simulink model "Dimmer"  (R2014a)
settings: Solver=ode15s  StartTime=0.0  StopTime=0.08  MaxStep=0.001  RelTol=1e-3
libraries: fl_lib x31, elec_lib x7, nesl_utility x4
Description:
  | Full-Wave Bridge Rectifier
  | 
  | This example shows an ideal AC transformer plus full-wave bridge rectifier.
  | It converts 120 volts AC to 12 volts DC. The transformer has a turns ratio
  | of 14, stepping the supply down to 8.6 volts rms, i.e. 8.6*sqrt(2) = 12 volts
  | pk-pk. The full-wave bridge rectifier plus capacitor combination
  | then converts this to DC. The resistor represents a typical load.
  | 
  | The model can be used to size the capacitor required for a specified load.
  | For a given size of capacitor, as the load resistance is increased, the ripple
  | in the DC voltage increases. The model can also be used to drive an
  | application circuit in order to assess the effect of the ripple.
  | 
  | 
  | 
  | 
  | Copyright 2008-2014 The MathWorks, Inc.
settings Model: ExtModeAutoUpdateStatusClock=off  Creator=MathWorks  LastModifiedBy=keelan
settings DataIOCC: SignalLoggingSaveFormat=ModelDataLogs
settings OptimizationCC: ExpressionDepthLimit=2147483647  InitFltsAndDblsToZero=on  EfficientMapNaN2IntZero=off
settings DebuggingCC: SaveWithParameterizedLinksMsg=none  UnderspecifiedInitializationDetection=Classic  SignalResolutionControl=TryResolveAllWithWarning  FcnCallInpInsideContextMsg=UseLocalSettings  StateNameClashWarn=warning
settings GRTTargetCC: TargetFcnLib=ansi_tfl_tmw.mat  CombineOutputUpdateFcns=off  GRTInterface=on
settings SimscapeCC: ExplicitSolverDiagnosticOptions=none

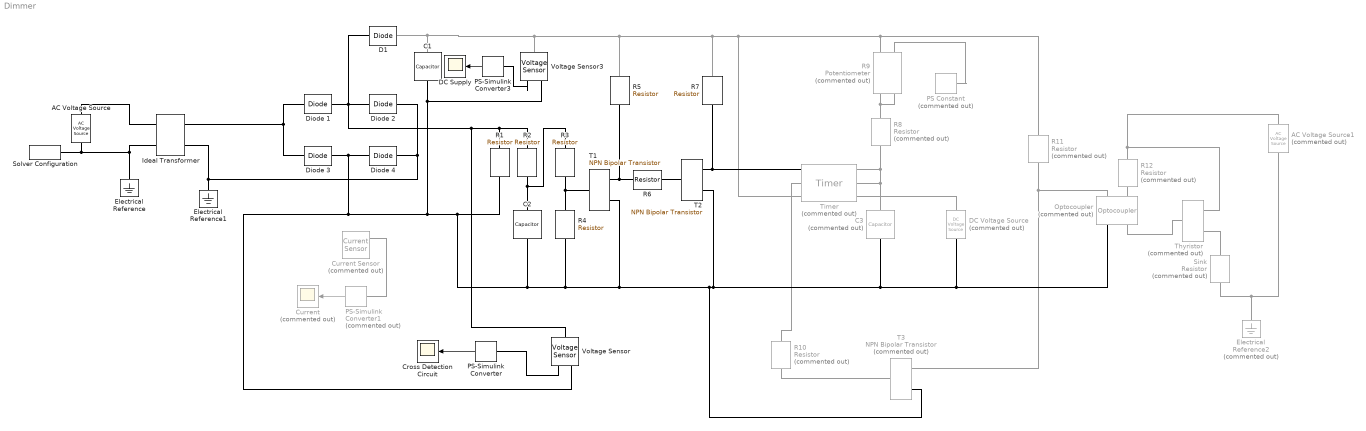
== system Dimmer ==
  AC Voltage Source : fl_lib/Electrical/Electrical Sources/AC Voltage Source  amp=240 V  shift=0 deg  frequency=50 Hz  omega=0 rad/s
  AC Voltage Source1 : fl_lib/Electrical/Electrical Sources/AC Voltage Source  Commented=on  amp=240 V  shift=0 deg  frequency=50 Hz  omega=0 rad/s
  C1 : fl_lib/Electrical/Electrical Elements/Capacitor  c=1000 uF  r=1e-06 Ohm  g=0 1/Ohm  i_specify=off  i_priority=High  i=0 A  v_specify=off  v_priority=High  v=0 V  vc_specify=on  vc_priority=High  vc=0 V
  C2 : fl_lib/Electrical/Electrical Elements/Capacitor  c=0.1 nF  r=1e-06 Ohm  g=0 1/Ohm  i_specify=off  i_priority=High  i=0 A  v_specify=off  v_priority=High  v=0 V  vc_specify=on  vc_priority=High  vc=0 V
  C3 : fl_lib/Electrical/Electrical Elements/Capacitor  Commented=on  c=1 uF  r=1e-06 Ohm  g=0 1/Ohm  i_specify=off  i_priority=High  i=0 A  v_specify=off  v_priority=High  v=0 V  vc_specify=on  vc_priority=High  vc=0 V
  Cross Detection Circuit : Scope
      settings: YMin=-0.25  YMax=3.5
  Current : Scope  Commented=on
      settings: YMin=-0.25  YMax=3.5
  Current Sensor : fl_lib/Electrical/Electrical Sensors/Current Sensor  Commented=on
  D1 : fl_lib/Electrical/Electrical Elements/Diode  Vf=0.1 V  Ron=0.1 Ohm  Goff=1e-8 1/Ohm  i_specify=off  i_priority=High  i=0 A  v_specify=off  v_priority=High  v=0 V
  DC Supply : Scope
      settings: TimeRange=10  YMin=-0.5  YMax=7.5  SaveName=ScopeData3
  DC Voltage Source : fl_lib/Electrical/Electrical Sources/DC Voltage Source  Commented=on  v0=0 V
  Diode {1..4} (4 alike) : fl_lib/Electrical/Electrical Elements/Diode  Vf=0.6 V  Ron=0.3 Ohm  Goff=1e-08 1/Ohm  i_specify=off  i_priority=High  i=0 A  v_specify=off  v_priority=High  v=0 V
  Electrical Reference : fl_lib/Electrical/Electrical Elements/Electrical Reference
  Electrical Reference1 : fl_lib/Electrical/Electrical Elements/Electrical Reference
  Electrical Reference2 : fl_lib/Electrical/Electrical Elements/Electrical Reference  Commented=on
  Ideal Transformer : fl_lib/Electrical/Electrical Elements/Ideal Transformer  n=26.666*2  i1_specify=off  i1_priority=High  i1=0 A  v1_specify=off  v1_priority=High  v1=0 V  i2_specify=off  i2_priority=High  i2=0 A  v2_specify=off  v2_priority=High  v2=0 V
  Optocoupler : elec_lib/Semiconductor Devices/Optocoupler  Commented=on  CTR=0.2  prmExp=1  I12=[ 0.001 0.015 ] A  V12=[ 0.9 1.05 ] V  RS=0.1 Ohm  IS=1e-10 A  Tmeas=25 C  ec=2  C_param=1  CJ0=5 pF  VJ=1 V  Mgrad=0.5  Vvec=[ 0.1 10 100 ] V  Cvec=[ 3.5 1 0.4 ] pF  FC=0.5  T_param=1  IS_T2=1.8e-8 A  I1_T2=0.029 A  V1_T2=1.05 V  Tmeas2=125 C  EG_param=1  EG=1.11 eV  XTI_param=1  XTI=3  Tdevice=25 C  Rth=[ 0 10 ] K/W  thermal_mass_parameterization=1  thermal_mass=[ 0 1 ] J/K  thermal_time_constant=[ 0 10 ] s  thermal_mass_initial_temperatures=[ 25 25 ] C
  PS Constant : fl_lib/Physical Signals/Sources/PS Constant  Commented=on  constant=1
  PS-Simulink Converter : nesl_utility/PS-Simulink Converter  PhysicalDomain=network_engine_domain  SubClassName=ps_output  LeftPortType=input  RightPortType=output  PseudoPeriodic=off  Frequencies=[]  Unit=1  AffineConversion=off
  PS-Simulink Converter1 : nesl_utility/PS-Simulink Converter  Commented=on  PhysicalDomain=network_engine_domain  SubClassName=ps_output  LeftPortType=input  RightPortType=output  PseudoPeriodic=off  Frequencies=[]  Unit=1  AffineConversion=off
  PS-Simulink Converter3 : nesl_utility/PS-Simulink Converter  PhysicalDomain=network_engine_domain  SubClassName=ps_output  LeftPortType=input  RightPortType=output  PseudoPeriodic=off  Frequencies=[]  Unit=1  AffineConversion=off
  R1 : fl_lib/Electrical/Electrical Elements/Resistor  R=10 kOhm  i_specify=off  i_priority=High  i=0 A  v_specify=off  v_priority=High  v=0 V
  R{8,10..12} (4 alike) : fl_lib/Electrical/Electrical Elements/Resistor  Commented=on  R=1 kOhm  i_specify=off  i_priority=High  i=0 A  v_specify=off  v_priority=High  v=0 V
  R2 : fl_lib/Electrical/Electrical Elements/Resistor  R=1 kOhm  i_specify=off  i_priority=High  i=0 A  v_specify=off  v_priority=High  v=0 V
  R3 : fl_lib/Electrical/Electrical Elements/Resistor  R=4.7 kOhm  i_specify=off  i_priority=High  i=0 A  v_specify=off  v_priority=High  v=0 V
  R4 : fl_lib/Electrical/Electrical Elements/Resistor  R=100 kOhm  i_specify=off  i_priority=High  i=0 A  v_specify=off  v_priority=High  v=0 V
  R5 : fl_lib/Electrical/Electrical Elements/Resistor  R=10 kOhm  i_specify=off  i_priority=High  i=0 A  v_specify=off  v_priority=High  v=0 V
  R6 : fl_lib/Electrical/Electrical Elements/Resistor  R=1 kOhm  i_specify=off  i_priority=High  i=0 A  v_specify=off  v_priority=High  v=0 V
  R7 : fl_lib/Electrical/Electrical Elements/Resistor  R=4.7 kOhm  i_specify=off  i_priority=High  i=0 A  v_specify=off  v_priority=High  v=0 V
  R9 : elec_lib/Passive Devices/Potentiometer  Commented=on  R0=100 kOhm  Rw=1 Ohm  Rcenter=200 Ohm  xmin=0  xmax=1  Taper=1  Gradient=1  xminL=0  xmaxL=1  lambda=1  A=1 Ohm
  Sink : fl_lib/Electrical/Electrical Elements/Resistor  Commented=on  R=0.1 kOhm  i_specify=off  i_priority=High  i=0 A  v_specify=off  v_priority=High  v=0 V
  Solver Configuration : nesl_utility/Solver Configuration  PhysicalDomain=network_engine_domain  SubClassName=solver  LeftPortType=input  RightPortType=generic  Accelerate=off  Tones=[]  Harmonics=[]  SimulateNoise=off  Profile=off  UseLocalSampling=off  EnableSwitchedLinearOptims=on  FrequencyDomain=off  UseCCode=off  RelTol=0.001  AbsTol=1e-06  MinStep=1e-09  ToWorkspace=off  DoDC=off  ResidualTolerance=1e-9  UseLocalSolver=off  LocalSolverChoice=NE_BACKWARD_EULER_ADVANCER  LocalSolverSampleTime=.001  DoFixedCost=off  MaxNonlinIter=3  MaxModeIter=2  LinearAlgebra=Sparse  DelaysMemoryBudget=1024  AutomaticFiltering=on  FilteringTimeConstant=0.001
  T1 : elec_lib/Semiconductor Devices/NPN Bipolar Transistor  parameterization=1  prmDatasheet=1  prmEquCoeff=1  BF=100  IS=1e-14 A  ec=1  VAF=200 V  hfe=100  hoe=5e-5 1/Ohm  Ic_h=100 mA  Vce_h=30 V  V1=0.55 V  I1=0.5 mA  BR=1  Tmeas=25 C  RC=0.01 Ohm  RE=1e-4 Ohm  RB=1 Ohm  C_BC=5 pF  C_BE=5 pF  TF=0 us  TR=0 us  hfe_T2=125  XTB=0  V1_T2=0.45 V  I1_T2=0.5 mA  Tmeas2=125 C  EG=1.11 eV  XTI=3  TdeviceDatasheet=25 C  TdeviceEquCoeff=25 C  Rth=[ 0 10 ] K/W  thermal_mass_parameterization=1  thermal_mass=[ 0 1 ] J/K  thermal_time_constant=[ 0 10 ] s  thermal_mass_initial_temperatures=[ 25 25 ] C
  T2 : elec_lib/Semiconductor Devices/NPN Bipolar Transistor  parameterization=1  prmDatasheet=1  prmEquCoeff=1  BF=100  IS=1e-14 A  ec=1  VAF=200 V  hfe=100  hoe=5e-5 1/Ohm  Ic_h=100 mA  Vce_h=30 V  V1=0.55 V  I1=0.5 mA  BR=1  Tmeas=25 C  RC=0.01 Ohm  RE=1e-4 Ohm  RB=1 Ohm  C_BC=5 pF  C_BE=5 pF  TF=0 us  TR=0 us  hfe_T2=125  XTB=0  V1_T2=0.45 V  I1_T2=0.5 mA  Tmeas2=125 C  EG=1.11 eV  XTI=3  TdeviceDatasheet=25 C  TdeviceEquCoeff=25 C  Rth=[ 0 10 ] K/W  thermal_mass_parameterization=1  thermal_mass=[ 0 1 ] J/K  thermal_time_constant=[ 0 10 ] s  thermal_mass_initial_temperatures=[ 25 25 ] C
  T3 : elec_lib/Semiconductor Devices/NPN Bipolar Transistor  Commented=on  parameterization=1  prmDatasheet=1  prmEquCoeff=1  BF=100  IS=1e-14 A  ec=1  VAF=200 V  hfe=100  hoe=5e-5 1/Ohm  Ic_h=100 mA  Vce_h=30 V  V1=0.55 V  I1=0.5 mA  BR=1  Tmeas=25 C  RC=0.01 Ohm  RE=1e-4 Ohm  RB=1 Ohm  C_BC=5 pF  C_BE=5 pF  TF=0 us  TR=0 us  hfe_T2=125  XTB=0  V1_T2=0.45 V  I1_T2=0.5 mA  Tmeas2=125 C  EG=1.11 eV  XTI=3  TdeviceDatasheet=25 C  TdeviceEquCoeff=25 C  Rth=[ 0 10 ] K/W  thermal_mass_parameterization=1  thermal_mass=[ 0 1 ] J/K  thermal_time_constant=[ 0 10 ] s  thermal_mass_initial_temperatures=[ 25 25 ] C
  Thyristor : elec_lib/Semiconductor Devices/Thyristor  Commented=on  model_type=1  v_on=1.2 V  i_on=1 A  VT_vec=[ 0.75 1 1.25 1.5 1.75 2 2.25 ] V  IT_vec=[ 0.015 0.22 0.75 1.4 2 2.75 3.45 ] A  IDRM=0.01 mA  VDRM=400 V  i_H=1 mA  Tmeas=25 C  i_GT=3 uA  v_GT=0.6 V  V_D=12 V  R=120 Ohm  dVdt=150 V/us  R_GK=1000 Ohm  TF_NPN_parameterization=1  T_d=2 us  i_d=10 mA  TF_NPN=0.3 us  TF_PNP_parameterization=1  TF_PNP=0.3 us  t_on_delay=0 s  t_on_curr=1 mA  t_on_rise=0 s  Rs=87 kOhm  Rgate=10 Ohm  Gain=10  Rth=[ 0 10 ] K/W  thermal_mass_parameterization=1  thermal_mass=[ 0 1 ] J/K  thermal_time_constant=[ 0 10 ] s  thermal_mass_initial_temperatures=[ 25 25 ] C
  Timer : elec_lib/Integrated Circuits/Timer  Commented=on  V_CC=7 V  V_OL=0 V  V_OH=7 V  R_OUT=8 Ohm  Delay=1e-7 s  R_DIV=5 kOhm  R_closed=12 Ohm  R_open=5e+8 Ohm
  Voltage Sensor : fl_lib/Electrical/Electrical Sensors/Voltage Sensor
  Voltage Sensor3 : fl_lib/Electrical/Electrical Sensors/Voltage Sensor
  wires:
  PS-Simulink Converter/1 -> Cross Detection Circuit/1
  PS-Simulink Converter3/1 -> DC Supply/1
  PS-Simulink Converter1/1 -> Current/1
  connections:
  Ideal Transformer/LConn2 -- AC Voltage Source/RConn1 -- Solver Configuration/RConn1 -- Electrical Reference/LConn1
  Ideal Transformer/LConn1 -- AC Voltage Source/LConn1
  Ideal Transformer/RConn1 -- Diode 3/RConn1 -- Diode 1/LConn1
  Diode 1/RConn1 -- R2/LConn1 -- R1/LConn1 -- Voltage Sensor/LConn1 -- D1/LConn1 -- Diode 2/RConn1
  Ideal Transformer/RConn2 -- Diode 2/LConn1 -- Diode 4/RConn1 -- Electrical Reference1/LConn1
  Voltage Sensor/RConn1 -- PS-Simulink Converter/LConn1
  R9/RConn1 -- R11/LConn1 -- Timer/LConn3 -- Voltage Sensor3/LConn1 -- D1/RConn1 -- C1/LConn1 -- R5/LConn1 -- R7/LConn1
  Voltage Sensor3/RConn1 -- PS-Simulink Converter3/LConn1
  C2/LConn1 -- R3/LConn1 -- R2/RConn1
  R3/RConn1 -- T1/LConn1 -- R4/LConn1
  T1/RConn1 -- R6/LConn1 -- R5/RConn1
  R6/RConn1 -- T2/LConn1
  T2/RConn1 -- Timer/LConn1 -- R7/RConn1
  R8/LConn1 -- R9/LConn2 -- R9/LConn1
  PS Constant/RConn1 -- R9/RConn2
  Timer/LConn2 -- R10/LConn1
  R10/RConn1 -- T3/LConn1
  T3/RConn1 -- Optocoupler/LConn1 -- R11/RConn1
  Optocoupler/LConn2 -- R12/RConn1
  AC Voltage Source1/LConn1 -- Thyristor/RConn1 -- R12/LConn1
  Sink/RConn1 -- Electrical Reference2/LConn1 -- AC Voltage Source1/RConn1
  Optocoupler/RConn2 -- Thyristor/LConn1
  Diode 3/LConn1 -- DC Voltage Source/RConn1 -- Optocoupler/RConn1 -- C3/RConn1 -- T2/RConn2 -- T3/RConn2 -- T1/RConn2 -- R4/RConn1 -- C2/RConn1 -- R1/RConn1 -- Voltage Sensor3/RConn2 -- C1/RConn1 -- Voltage Sensor/RConn2 -- Diode 4/LConn1
  DC Voltage Source/LConn1 -- Timer/RConn3
  Timer/RConn2 -- C3/LConn1 -- Timer/RConn1 -- R8/RConn1
  Thyristor/RConn2 -- Sink/LConn1
  Current Sensor/RConn1 -- PS-Simulink Converter1/LConn1
